simulink model "dds_taylor_corrected"  (R2016b)
settings: Solver=VariableStepAuto  StartTime=0.0  StopTime=1e5  RelTol=1e-3  EnableMultiTasking=on
undefined symbols (not defined in the file): Fadc
libraries: xbsIndex_r4 x71
settings Model: Creator=Mitch  LastModifiedBy=mdewart
settings OptimizationCC: LifeSpan=inf
settings DebuggingCC: SFUnexpectedBacktrackingDiag=warning  SFNoUnconditionalDefaultTransitionDiag=warning  SFExecutionAtInitializationDiag=none
settings GRTTargetCC: TargetLangStandard=C89/C90 (ANSI)  GeneratePreprocessorConditionals=Disable all
settings ConfigComp: CovMetricSettings=dw  CovHtmlReporting=on  CovSaveCumulativeToWorkspaceVar=on  CovSaveSingleToWorkspaceVar=on  CovExternalEMLEnable=off

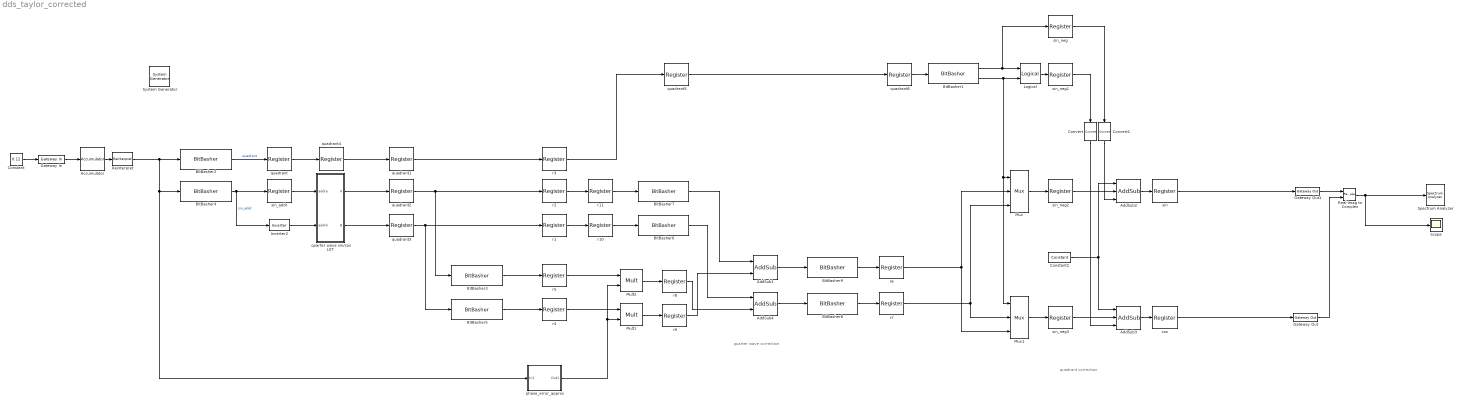
== system dds_taylor_corrected ==
  note: quadrant correction
  note: quarter wave correction
  " System Generator" : xbsIndex_r4/ System Generator  Tag=genX  xilinxfamily=kintexu  part=xcku060  speed=-2-e  package=ffva1156  synthesis_tool=Vivado  clock_wrapper=Clock Enables  directory=./netlist2  proj_type=Vivado  Synth_file=Vivado Synthesis Defaults  Impl_file=Vivado Implementation Defaults  testbench=off  simulink_period=2/Fadc  sysclk_period=2e9/Fadc  dcm_input_clock_period=10  incr_netlist=off  trim_vbits=Everywhere in SubSystem  dbl_ovrd=According to Block Masks  core_generation=According to Block Masks  run_coregen=off  deprecated_control=off  eval_field=0  block_type=sysgen
  Accumulator : xbsIndex_r4/Accumulator  operation=Add  n_bits=20  overflow=Wrap  scale=1  rst=off  hasbypass=off  infoeditControl=reset for floating point data type must be asserted for a minimum of 2 cycles  en=off  latency=1  msb_inp=100  msb=100  lsb=-100  use_behavioral_HDL=on  implementation=Fabric  dbl_ovrd=off  block_type=accum
  AddSub1 : xbsIndex_r4/AddSub  mode=Addition  use_carryin=off  use_carryout=off  en=off  latency=0  precision=Full  arith_type="Signed  (2's comp)"  n_bits=18  bin_pt=0  quantization=Truncate  overflow=Wrap  use_behavioral_HDL=on  hw_selection=Fabric  pipelined=off  dbl_ovrd=off  block_type=addsub
  AddSub2 : xbsIndex_r4/AddSub  mode=Addition or Subtraction  use_carryin=off  use_carryout=off  en=off  latency=0  precision=Full  arith_type="Signed  (2's comp)"  n_bits=18  bin_pt=17  quantization=Truncate  overflow=Wrap  use_behavioral_HDL=on  hw_selection=Fabric  pipelined=off  dbl_ovrd=off  block_type=addsub
  AddSub3 : xbsIndex_r4/AddSub  mode=Addition or Subtraction  use_carryin=off  use_carryout=off  en=off  latency=0  precision=Full  arith_type="Signed  (2's comp)"  n_bits=18  bin_pt=17  quantization=Truncate  overflow=Wrap  use_behavioral_HDL=on  hw_selection=Fabric  pipelined=off  dbl_ovrd=off  block_type=addsub
  AddSub4 : xbsIndex_r4/AddSub  mode=Subtraction  use_carryin=off  use_carryout=off  en=off  latency=0  precision=Full  arith_type="Signed  (2's comp)"  n_bits=18  bin_pt=0  quantization=Truncate  overflow=Wrap  use_behavioral_HDL=on  hw_selection=Fabric  pipelined=off  dbl_ovrd=off  block_type=addsub
  BitBasher1 : xbsIndex_r4/BitBasher  bitexpr=|  display_expr=on  sr_1=out1  arith_type1=Unsigned  bin_pt1=0  sr_2=out0  arith_type2=Unsigned  bin_pt2=0  sr_3=3  arith_type3=Unsigned  bin_pt3=0  sr_4=4  arith_type4=Unsigned  bin_pt4=0  dbl_ovrd=off  block_type=bitbasher
      | out1 = {in[1]}
      | out0 = {in[0]}
  BitBasher2 : xbsIndex_r4/BitBasher  bitexpr=out={in[19:18]}  display_expr=on  sr_1=out  arith_type1=Unsigned  bin_pt1=0  sr_2=b  arith_type2=Unsigned  bin_pt2=0  sr_3=3  arith_type3=Unsigned  bin_pt3=0  sr_4=4  arith_type4=Unsigned  bin_pt4=0  dbl_ovrd=off  block_type=bitbasher
  BitBasher3 : xbsIndex_r4/BitBasher  bitexpr=out={1'b0,in[17:8]}  display_expr=on  sr_1=out  arith_type1="Signed  (2's comp)"  bin_pt1=0  sr_2=table_width-1 downto  arith_type2=Unsigned  bin_pt2=0  sr_3=3  arith_type3=Unsigned  bin_pt3=0  sr_4=4  arith_type4=Unsigned  bin_pt4=0  dbl_ovrd=off  block_type=bitbasher
  BitBasher4 : xbsIndex_r4/BitBasher  bitexpr=out={in[17:8]}  display_expr=on  sr_1=out  arith_type1=Unsigned  bin_pt1=0  sr_2=b  arith_type2=Unsigned  bin_pt2=0  sr_3=3  arith_type3=Unsigned  bin_pt3=0  sr_4=4  arith_type4=Unsigned  bin_pt4=0  dbl_ovrd=off  block_type=bitbasher
  BitBasher5 : xbsIndex_r4/BitBasher  bitexpr=out={1'b0,in[17:8]}  display_expr=on  sr_1=out  arith_type1="Signed  (2's comp)"  bin_pt1=0  sr_2=table_width-1 downto  arith_type2=Unsigned  bin_pt2=0  sr_3=3  arith_type3=Unsigned  bin_pt3=0  sr_4=4  arith_type4=Unsigned  bin_pt4=0  dbl_ovrd=off  block_type=bitbasher
  BitBasher6 : xbsIndex_r4/BitBasher  bitexpr=out={1'b0,in,11'b1}  display_expr=on  sr_1=out  arith_type1="Signed  (2's comp)"  bin_pt1=0  sr_2=table_width-1 downto  arith_type2=Unsigned  bin_pt2=0  sr_3=3  arith_type3=Unsigned  bin_pt3=0  sr_4=4  arith_type4=Unsigned  bin_pt4=0  dbl_ovrd=off  block_type=bitbasher
  BitBasher7 : xbsIndex_r4/BitBasher  bitexpr=out={1'b0,in,11'b1}  display_expr=on  sr_1=out  arith_type1="Signed  (2's comp)"  bin_pt1=0  sr_2=table_width-1 downto  arith_type2=Unsigned  bin_pt2=0  sr_3=3  arith_type3=Unsigned  bin_pt3=0  sr_4=4  arith_type4=Unsigned  bin_pt4=0  dbl_ovrd=off  block_type=bitbasher
  BitBasher8 : xbsIndex_r4/BitBasher  bitexpr=out1 = {in[28:11]}  display_expr=on  sr_1=out1  arith_type1="Signed  (2's comp)"  bin_pt1=17  sr_2=out0  arith_type2=Unsigned  bin_pt2=0  sr_3=3  arith_type3=Unsigned  bin_pt3=0  sr_4=4  arith_type4=Unsigned  bin_pt4=0  dbl_ovrd=off  block_type=bitbasher
  BitBasher9 : xbsIndex_r4/BitBasher  bitexpr=out1 = {in[28:11]}  display_expr=on  sr_1=out1  arith_type1="Signed  (2's comp)"  bin_pt1=17  sr_2=out0  arith_type2=Unsigned  bin_pt2=0  sr_3=3  arith_type3=Unsigned  bin_pt3=0  sr_4=4  arith_type4=Unsigned  bin_pt4=0  dbl_ovrd=off  block_type=bitbasher
  Constant : Constant  Value=0.12
  Constant2 : xbsIndex_r4/Constant  const=0  gui_display_data_type=Fixed-point  arith_type=Unsigned  n_bits=1  bin_pt=0  preci_type=Single  exp_width=8  frac_width=24  explicit_period=off  period=1  equ=P=C  opselect=C  inp2=PCIN>>17  opr=+  inp1=P  carry=CIN  dbl_ovrd=off  block_type=constant
  Convert : xbsIndex_r4/Convert  gui_display_data_type=Boolean  arith_type=Boolean  n_bits=16  bin_pt=14  float_type=Single  exp_bits=8  fraction_bits=24  quantization=Truncate  overflow=Wrap  en=off  latency=0  pipeline=off  dbl_ovrd=off  block_type=convert
  Convert1 : xbsIndex_r4/Convert  gui_display_data_type=Boolean  arith_type=Boolean  n_bits=16  bin_pt=14  float_type=Single  exp_bits=8  fraction_bits=24  quantization=Truncate  overflow=Wrap  en=off  latency=0  pipeline=off  dbl_ovrd=off  block_type=convert
  Gateway In : xbsIndex_r4/Gateway In  gui_display_data_type=Fixed-point  arith_type=Unsigned  n_bits=20  bin_pt=20  preci_type=Single  exp_width=8  frac_width=24  rows=1  columns=1  quantization="Round  (unbiased: +/- Inf)"  overflow=Saturate  period=2/Fadc  UseAsADC=off  ADCChannel='1'  interface=None  automatic_assignment=on  address_offset=hex2dec('00')  intf_name=''  intf_description=''  default_value=0  timing_constraint=None  locs_specified=off  LOCs={}  io_standard={}  inherit_from_input=off  hdl_port=on  dbl_ovrd=off  block_type=gatewayin
  Gateway Out : xbsIndex_r4/Gateway Out  inherit_from_input=off  hdl_port=on  rows=1  columns=1  UseAsDAC=off  DACChannel='1'  interface=None  automatic_assignment=on  address_offset=hex2dec('00')  intf_name=''  intf_description=''  timing_constraint=None  locs_specified=off  LOCs={}  io_standard={}  block_type=gatewayout
  Gateway Out1 : xbsIndex_r4/Gateway Out  inherit_from_input=off  hdl_port=on  rows=1  columns=1  UseAsDAC=off  DACChannel='1'  interface=None  automatic_assignment=on  address_offset=hex2dec('00')  intf_name=''  intf_description=''  timing_constraint=None  locs_specified=off  LOCs={}  io_standard={}  block_type=gatewayout
  Inverter2 : xbsIndex_r4/Inverter  en=off  latency=1  dbl_ovrd=off  block_type=inv
  Logical : xbsIndex_r4/Logical  logical_function=XOR  inputs=2  en=off  latency=0  precision=Full  arith_type=Unsigned  n_bits=16  bin_pt=0  align_bp=on  dbl_ovrd=off  block_type=logical
  Mult1 : xbsIndex_r4/Mult  precision=Full  arith_type="Signed  (2's comp)"  n_bits=21  bin_pt=0  quantization=Truncate  overflow=Wrap  en=off  latency=0  use_behavioral_HDL=on  opt=Speed  use_embedded=on  optimum_pipeline=off  pipeline=on  dbl_ovrd=off  use_rpm=on  placement_style=Triangular  block_type=mult
  Mult2 : xbsIndex_r4/Mult  precision=Full  arith_type="Signed  (2's comp)"  n_bits=21  bin_pt=0  quantization=Truncate  overflow=Wrap  en=off  latency=0  use_behavioral_HDL=on  opt=Speed  use_embedded=on  optimum_pipeline=off  pipeline=on  dbl_ovrd=off  use_rpm=on  placement_style=Triangular  block_type=mult
  Mux : xbsIndex_r4/Mux  inputs=2  en=off  latency=0  precision=Full  arith_type=Unsigned  n_bits=16  bin_pt=14  quantization=Truncate  overflow=Wrap  dbl_ovrd=off  block_type=mux
  Mux1 : xbsIndex_r4/Mux  inputs=2  en=off  latency=0  precision=Full  arith_type=Unsigned  n_bits=16  bin_pt=14  quantization=Truncate  overflow=Wrap  dbl_ovrd=off  block_type=mux
  Real-Imag to Complex : RealImagToComplex
  Reinterpret : xbsIndex_r4/Reinterpret  force_arith_type=on  arith_type=Unsigned  force_bin_pt=on  bin_pt=0  block_type=reinterpret
  Scope : Scope
  Spectrum Analyzer : SpectrumAnalyzer
  cos : xbsIndex_r4/Register  init=0  rst=off  en=off  dbl_ovrd=off  block_type=register
  phase_error_approx : Subsystem
  quadrant{,1..5,8} (7 alike) : xbsIndex_r4/Register  init=0  rst=off  en=off  dbl_ovrd=off  block_type=register
  quarter wave sin/cos LUT : Subsystem
  r{1..11} (11 alike) : xbsIndex_r4/Register  init=0  rst=off  en=off  dbl_ovrd=off  block_type=register
  sin : xbsIndex_r4/Register  init=0  rst=off  en=off  dbl_ovrd=off  block_type=register
  sin_addr : xbsIndex_r4/Register  init=0  rst=off  en=off  dbl_ovrd=off  block_type=register
  sin_neg{,1..3} (4 alike) : xbsIndex_r4/Register  init=0  rst=off  en=off  dbl_ovrd=off  block_type=register
  wires:
  Gateway Out1/1 -> Real-Imag to Complex/1
  Gateway Out/1 -> Real-Imag to Complex/2
  Real-Imag to Complex/1 -> Scope/1, Spectrum Analyzer/1
  Constant/1 -> Gateway In/1
  Accumulator/1 -> Reinterpret/1
  Gateway In/1 -> Accumulator/1
  Convert1/1 -> AddSub2/3
  Inverter2/1 -> quarter wave sin/cos LUT/2(addrb)
  phase_error_approx/1(Out1) -> Mult2/2, Mult1/2
  Mux1/1 -> sin_neg3/1
  sin_neg2/1 -> AddSub2/2
  BitBasher3/1 -> r5/1
  Mult1/1 -> r9/1
  sin_neg1/1 -> Convert/1
  quadrant1/1 -> r3/1
  cos/1 -> Gateway Out/1
  quadrant/1 -> quadrant4/1
  BitBasher2/1 -> quadrant/1  "quadrant"
  Mux/1 -> sin_neg2/1
  BitBasher9/1 -> r6/1
  quadrant4/1 -> quadrant1/1
  r7/1 -> Mux/3, Mux1/2
  AddSub1/1 -> BitBasher9/1
  AddSub4/1 -> BitBasher8/1
  BitBasher8/1 -> r7/1
  r6/1 -> Mux1/3, Mux/2
  quadrant5/1 -> quadrant8/1
  Mult2/1 -> r8/1
  quadrant2/1 -> BitBasher3/1, r2/1
  BitBasher5/1 -> r4/1
  quarter wave sin/cos LUT/2(B) -> quadrant3/1
  BitBasher6/1 -> AddSub4/1
  sin_neg3/1 -> AddSub3/2
  AddSub3/1 -> cos/1
  r8/1 -> AddSub4/2
  r2/1 -> r11/1
  AddSub2/1 -> sin/1
  Logical/1 -> sin_neg1/1
  Convert/1 -> AddSub3/3
  sin_addr/1 -> quarter wave sin/cos LUT/1(addra)
  r1/1 -> r10/1
  r5/1 -> Mult2/1
  r9/1 -> AddSub1/2
  BitBasher7/1 -> AddSub1/1
  BitBasher4/1 -> Inverter2/1, sin_addr/1  "sin_addr"
  r4/1 -> Mult1/1
  quadrant3/1 -> BitBasher5/1, r1/1
  BitBasher1/1 -> Logical/1, sin_neg/1
  BitBasher1/2 -> Logical/2, Mux/1, Mux1/1
  sin_neg/1 -> Convert1/1
  Constant2/1 -> AddSub2/1, AddSub3/1
  quarter wave sin/cos LUT/1(A) -> quadrant2/1
  r3/1 -> quadrant5/1
  Reinterpret/1 -> phase_error_approx/1(In1), BitBasher4/1, BitBasher2/1
  quadrant8/1 -> BitBasher1/1
  sin/1 -> Gateway Out1/1
  r10/1 -> BitBasher6/1
  r11/1 -> BitBasher7/1

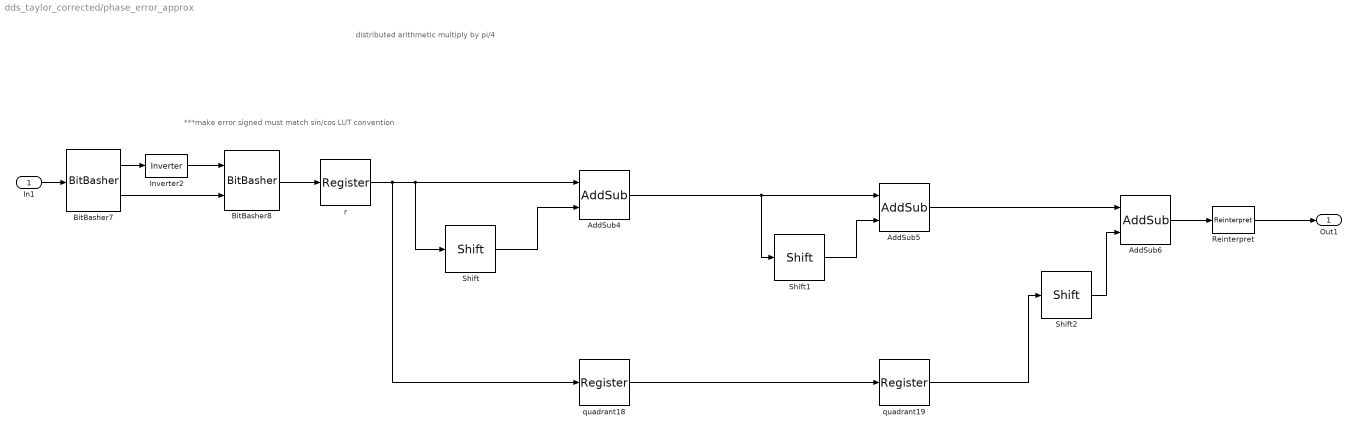
== system dds_taylor_corrected/phase_error_approx ==
  note: ***make error signed must match sin/cos LUT convention
  note: distributed arithmetic multiply by pi/4
  In1 : Inport
  AddSub4 : xbsIndex_r4/AddSub  mode=Addition  use_carryin=off  use_carryout=off  en=off  latency=1  precision=User Defined  arith_type="Signed  (2's comp)"  n_bits=10  bin_pt=9  quantization="Round  (unbiased: +/- Inf)"  overflow=Wrap  use_behavioral_HDL=on  hw_selection=Fabric  pipelined=off  dbl_ovrd=off  block_type=addsub
  AddSub5 : xbsIndex_r4/AddSub  mode=Addition  use_carryin=off  use_carryout=off  en=off  latency=1  precision=User Defined  arith_type="Signed  (2's comp)"  n_bits=10  bin_pt=9  quantization="Round  (unbiased: +/- Inf)"  overflow=Wrap  use_behavioral_HDL=on  hw_selection=Fabric  pipelined=off  dbl_ovrd=off  block_type=addsub
  AddSub6 : xbsIndex_r4/AddSub  mode=Addition  use_carryin=off  use_carryout=off  en=off  latency=1  precision=User Defined  arith_type="Signed  (2's comp)"  n_bits=10  bin_pt=9  quantization="Round  (unbiased: +/- Inf)"  overflow=Wrap  use_behavioral_HDL=off  hw_selection=Fabric  pipelined=off  dbl_ovrd=off  block_type=addsub
  BitBasher7 : xbsIndex_r4/BitBasher  bitexpr=|  display_expr=off  sr_1=a  arith_type1=Unsigned  bin_pt1=0  sr_2=b  arith_type2=Unsigned  bin_pt2=0  sr_3=3  arith_type3=Unsigned  bin_pt3=0  sr_4=4  arith_type4=Unsigned  bin_pt4=0  dbl_ovrd=off  block_type=bitbasher
      | a={in[7]}
      | b={in[6:0]}
  BitBasher8 : xbsIndex_r4/BitBasher  bitexpr=out = {sign, val}  display_expr=off  sr_1=out  arith_type1="Signed  (2's comp)"  bin_pt1=8  sr_2=b  arith_type2=Unsigned  bin_pt2=0  sr_3=3  arith_type3=Unsigned  bin_pt3=0  sr_4=4  arith_type4=Unsigned  bin_pt4=0  dbl_ovrd=off  block_type=bitbasher
  Inverter2 : xbsIndex_r4/Inverter  en=off  latency=0  dbl_ovrd=off  block_type=inv
  Reinterpret : xbsIndex_r4/Reinterpret  force_arith_type=on  arith_type="Signed  (2's comp)"  force_bin_pt=on  bin_pt=0  block_type=reinterpret
  Shift : xbsIndex_r4/Shift  shift_dir=Right  shift_bits=4  en=off  latency=0  precision=User Defined  arith_type="Signed  (2's comp)"  n_bits=10  bin_pt=10  quantization=Truncate  overflow=Wrap  dbl_ovrd=off  block_type=shift
  Shift1 : xbsIndex_r4/Shift  shift_dir=Right  shift_bits=7  en=off  latency=0  precision=User Defined  arith_type="Signed  (2's comp)"  n_bits=10  bin_pt=10  quantization=Truncate  overflow=Wrap  dbl_ovrd=off  block_type=shift
  Shift2 : xbsIndex_r4/Shift  shift_dir=Right  shift_bits=1  en=off  latency=0  precision=User Defined  arith_type="Signed  (2's comp)"  n_bits=9  bin_pt=9  quantization=Truncate  overflow=Wrap  dbl_ovrd=off  block_type=shift
  quadrant18 : xbsIndex_r4/Register  init=0  rst=off  en=off  dbl_ovrd=off  block_type=register
  quadrant19 : xbsIndex_r4/Register  init=0  rst=off  en=off  dbl_ovrd=off  block_type=register
  r : xbsIndex_r4/Register  init=0  rst=off  en=off  dbl_ovrd=off  block_type=register
  Out1 : Outport
  wires:
  AddSub4/1 -> Shift1/1, AddSub5/1
  Shift2/1 -> AddSub6/2
  AddSub5/1 -> AddSub6/1
  quadrant18/1 -> quadrant19/1
  Shift/1 -> AddSub4/2
  Shift1/1 -> AddSub5/2
  r/1 -> AddSub4/1, Shift/1, quadrant18/1
  BitBasher7/2 -> BitBasher8/2
  Inverter2/1 -> BitBasher8/1
  BitBasher8/1 -> r/1
  BitBasher7/1 -> Inverter2/1
  quadrant19/1 -> Shift2/1
  AddSub6/1 -> Reinterpret/1
  In1/1 -> BitBasher7/1
  Reinterpret/1 -> Out1/1

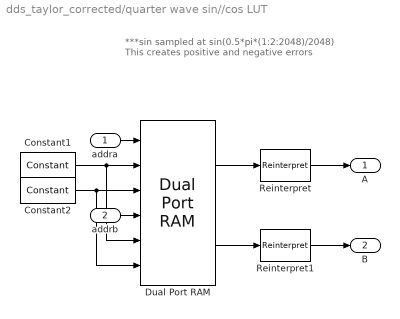
== system dds_taylor_corrected/quarter wave sin//cos LUT ==
  note: ***sin sampled at sin(0.5*pi*(1:2:2048)/2048)
      | This creates positive and negative errors
  addra : Inport
  addrb : Inport  Port=2
  Constant1 : xbsIndex_r4/Constant  const=0  gui_display_data_type=Fixed-point  arith_type=Unsigned  n_bits=18  bin_pt=17  preci_type=Single  exp_width=8  frac_width=24  explicit_period=off  period=1  equ=P=C  opselect=C  inp2=PCIN>>17  opr=+  inp1=P  carry=CIN  dbl_ovrd=off  block_type=constant
  Constant2 : xbsIndex_r4/Constant  const=0  gui_display_data_type=Boolean  arith_type=Boolean  n_bits=1  bin_pt=0  preci_type=Single  exp_width=8  frac_width=24  explicit_period=off  period=1  equ=P=C  opselect=C  inp2=PCIN>>17  opr=+  inp1=P  carry=CIN  dbl_ovrd=off  block_type=constant
  Dual Port RAM : xbsIndex_r4/Dual Port RAM  depth=1024  initVector=0.999*sin(0.5*pi*(1:2:2048)/2048)  distributed_mem=Block RAM  init_a=0  init_b=0  rst_a=off  rst_b=off  en_a=off  en_b=off  latency=1  write_mode_A=Read After Write  write_mode_B=Read After Write  optimize=Area  dbl_ovrd=off  block_type=dpram
  Reinterpret : xbsIndex_r4/Reinterpret  force_arith_type=on  arith_type=Unsigned  force_bin_pt=on  bin_pt=0  block_type=reinterpret
  Reinterpret1 : xbsIndex_r4/Reinterpret  force_arith_type=on  arith_type=Unsigned  force_bin_pt=on  bin_pt=0  block_type=reinterpret
  A : Outport
  B : Outport  Port=2
  wires:
  Constant1/1 -> Dual Port RAM/5, Dual Port RAM/2
  Dual Port RAM/2 -> Reinterpret1/1
  addra/1 -> Dual Port RAM/1
  Dual Port RAM/1 -> Reinterpret/1
  addrb/1 -> Dual Port RAM/4
  Constant2/1 -> Dual Port RAM/6, Dual Port RAM/3
  Reinterpret/1 -> A/1
  Reinterpret1/1 -> B/1
